simulink model "BLDC_FOC"  (R2020a)
settings: Solver=VariableStepAuto  StartTime=0.0  StopTime=2  RelTol=1e-3
InitFcn:
  | BLDC_FOC_Params
model workspace (MAT data in the model file):
  PhaseInductance = 0.001
  PhaseResistance = Simulink.Parameter
  PhaseResistance.Value = 0.03
  PhaseResistance.DataType = 'auto'
  PhaseResistance.Dimensions = [1 1]
values from neighbouring files (symbols this model uses):
  AlignmentDuration = 3 * TimeConstant_s    (= 0.2025)    [BLDC_FOC_Params.m]
  BatteryCapacityAh = 1.4    [BLDC_FOC_Params.m]
  BatteryCRating = 70    [BLDC_FOC_Params.m]
  BatteryVoltage = 1    [BLDC_FOC_Params.m]
  MaxCurrentDraw = (BatteryCapacityAh * BatteryCRating)/MotorCount    (= 98)    [BLDC_FOC_Params.m]
  MinimalOpenLoopSpeed_rpm = 100    [BLDC_FOC_Params.m]
  MotorCount = 1    [BLDC_FOC_Params.m]
  MotorKt = 0.00506    [BLDC_FOC_Params.m]
  MotorKv = 1890    [BLDC_FOC_Params.m]
  MotorPolePairs = 4    [BLDC_FOC_Params.m]
  MotorStatorTeeth = 0    [BLDC_FOC_Params.m]
  NominalTorque_Nm = 0.00183    [BLDC_FOC_Params.m]
  PhaseResistance_Ohm = DeltaToPhase(TerminalResistance_Ohm)    [BLDC_FOC_Params.m]
  PhaseSelfInductance_H = DeltaToPhase(TerminalInductance_H)    [BLDC_FOC_Params.m]
  RotorInertia_KgM2 = 0.00000011    (= 1.1e-07)    [BLDC_FOC_Params.m]
  Svpwm_freq_hz = 20000    [BLDC_FOC_Params.m]
undefined symbols (not defined in the file or in its folder): Down, Up
libraries: ee_lib x19, nesl_utility x14, fl_lib x12, eeTransforms x4, simulink x2, eePwmGenerator x1, powerlib_meascontrol x1
settings Model: Creator=enzoe  LastModifiedBy=enzoe

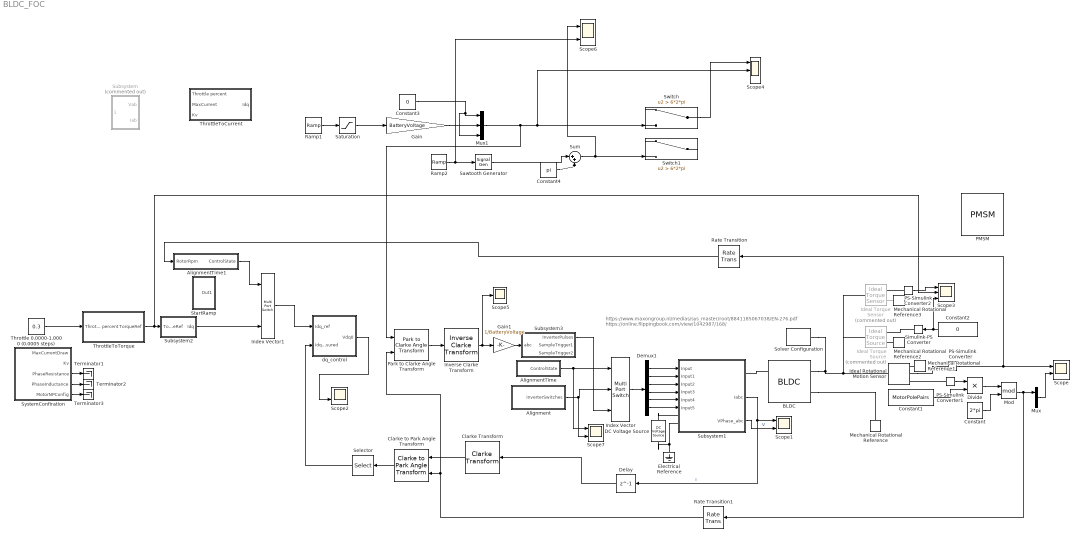
== system BLDC_FOC ==
  note: https://www.maxongroup.nl/medias/sys_master/root/8841185067038/EN-276.pdf
      | https://online.flippingbook.com/view/1042987/168/
  Alignment : Subsystem
  AlignmentTime : Subsystem
  AlignmentTime1 : Subsystem
  BLDC : ee_lib/Electromechanical/Permanent Magnet/BLDC  winding_type=ee.enum.statorconnection.wye  rotor_param=2  pm_flux_linkage=MaximumPermanentMagnetFluxLinkage Wb  theta_constant=pi / (MotorPolePairs*2) rad  emf_max=MaximumRotorInducedBackEmf_V V  DphiDtheta_tab=[0, -.1528, -.1528, .1528, .1528, 0] Wb/rad  back_emf_tab=[0, -9.6, -9.6, 9.6, 9.6, 0] V  rotor_angle_tab=[0, 7.5, 22.5, 37.5, 52.5, 60] deg  w_meas=RotorSpeedUsedForBackEmfMeasurement_RPM rpm  nPolePairs=MotorPolePairs  stator_param=ee.enum.statorparam.LsLmMs  machine_param=ee.enum.dqparameterization.constant  Ld=PhaseInductance H  Lq=PhaseInductance H  idVec=[-200, 0, 200] A  iqVec=[-200, 0, 200] A  LdMatrix=0.00022 * ones(3, 3) H  LqMatrix=0.00022 * ones(3, 3) H  L0=0.00016 H  Ls=PhaseSelfInductance_H H  Lm=StatorInductanceFluctuation_H H  Ms=StatorMutualInductance_H H  Rs=PhaseResistance_Ohm Ohm  zero_sequence=ee.enum.park.zerosequence.include  J=RotorInertia_KgM2 kg*m^2  lam=RotorDamping_NmRads N*m/(rad/s)  axes_param=2  i_d_specify=off  i_d_priority=None  i_d=0 A  i_d_nominal_specify=off  i_d_nominal_unit=A  i_d_nominal_value=1  i_q_specify=off  i_q_priority=None  i_q=0 A  i_q_nominal_specify=off  i_q_nominal_unit=A  i_q_nominal_value=1  torque_specify=off  torque_priority=None  torque=0 N*m  torque_nominal_specify=off  torque_nominal_unit=N*m  torque_nominal_value=1  angular_velocity_specify=off  angular_velocity_priority=High  angular_velocity=0 rpm  angular_velocity_nominal_specify=off  angular_velocity_nominal_unit=rpm  angular_velocity_nominal_value=1  angular_position_specify=off  angular_position_priority=High  angular_position=0 deg  angular_position_nominal_specify=off  angular_position_nominal_unit=deg  angular_position_nominal_value=1  loss_param=ee.enum.ironloss.none  losses_oc=[0, 0, 0] W  losses_sc=[0, 0, 0] W  f_losses=60 Hz  Isc_losses=95 A  Tmeas=298.15 K  alpha=3.93e-3 1/K  alpha_flux=-0.001 1/K  stator_thermal_mass=100 J/K  rotor_thermal_mass=200 J/K  Rm_percent_rotor=90  Rd_percent_rotor=30  temperatureA_specify=off  temperatureA_priority=High  temperatureA=25 degC  temperatureA_nominal_specify=off  temperatureA_nominal_unit=degC  temperatureA_nominal_value=1  temperatureB_specify=off  temperatureB_priority=High  temperatureB=25 degC  temperatureB_nominal_specify=off  temperatureB_nominal_unit=degC  temperatureB_nominal_value=1  temperatureC_specify=off  temperatureC_priority=High  temperatureC=25 degC  temperatureC_nominal_specify=off  temperatureC_nominal_unit=degC  temperatureC_nominal_value=1  temperatureR_specify=off  temperatureR_priority=High  temperatureR=25 degC  temperatureR_nominal_specify=off  temperatureR_nominal_unit=degC  temperatureR_nominal_value=1
      settings: SourceProductBaseCode=PS  InternalSimscapePortConfiguration="{\"Bottom\":[],\"Left\":[{\"id\":\"N\",\"label\":\"~\",\"type\":\"foundation.electrical.three_phase\"},{\"id\":\"n\",\"label\":\"n\",\"type\":\"foundation.electrical.electrical\"}],\"Right\":[{\"id\":\"R\",\"label\":\"R\",\"type\":\"foundation.mechanical.rotational.rotational\"},{\"id\":\"C\",\"label\":\"C\",\"type\":\"foundation.mechanical.rotational.rotational\"}],\"Top\":[]}"
  Clarke Transform : eeTransforms/Clarke Transform  PowerInvariant=off
      settings: SourceProductBaseCode=PS
  Clarke to Park Angle Transform : eeTransforms/Clarke to Park Angle Transform  AxisAlignment=D-axis
      settings: SourceProductBaseCode=PS
  Constant : Constant  Value=2*pi
  Constant1 : Constant  Value=MotorPolePairs
  Constant2 : Constant  Value=0
  Constant3 : Constant  Value=0
  Constant4 : Constant  Value=pi
  DC Voltage Source : ee_lib/Additional Components/SPICE Sources/DC Voltage Source  DC=BatteryVoltage V
  Delay : Delay  DelayLength=1
  Demux1 : Demux  Outputs=6
  Divide : Product  Inputs=**
  Electrical Reference : fl_lib/Electrical/Electrical Elements/Electrical Reference
  Gain : Gain  Gain=BatteryVoltage
  Gain1 : Gain  Gain=1/BatteryVoltage
  Ideal Rotational Motion Sensor : fl_lib/Mechanical/Mechanical Sensors/Ideal Rotational Motion Sensor  wrap_angle=simscape.enum.onoff.off  offset=0 rad
  Ideal Torque Sensor : fl_lib/Mechanical/Mechanical Sensors/Ideal Torque Sensor  Commented=on
  Ideal Torque Source : fl_lib/Mechanical/Mechanical Sources/Ideal Torque Source  Commented=on
  Index Vector : MultiPortSwitch  DataPortOrder=Zero-based contiguous  Inputs=2  zeroidx=on
  Index Vector1 : MultiPortSwitch  DataPortOrder=Zero-based contiguous  Inputs=2  zeroidx=on
  Inverse Clarke Transform : eeTransforms/Inverse Clarke Transform  PowerInvariant=off
      settings: SourceProductBaseCode=PS
  Mechanical Rotational Reference{,1..3} (4 alike) : fl_lib/Mechanical/Rotational Elements/Mechanical Rotational Reference
  Mod : Math  Operator=mod  SaturateOnIntegerOverflow=on
  Mux : Mux  Inputs=2
  Mux1 : Mux  Inputs=3
  PMSM : ee_lib/Electromechanical/Permanent Magnet/PMSM  winding_type=ee.enum.statorconnection.wye  machine_param=ee.enum.pmsm.parameterization.constant  nPolePairs=MotorPolePairs  pmflux_param=ee.enum.pmflux.backemfconstant  pm_flux_linkage=0.03 Wb  torque_constant=0.18 N*m/A  back_emf_constant=BackEmfConstant_VRpm V/rpm  stator_param=ee.enum.statorparam.LsLmMs  Ld=0.00019 H  Lq=0.00025 H  idVec=[-200, 0, 200] A  iqVec=[-200, 0, 200] A  LdMatrix=0.0002 * ones(3, 3) H  LqMatrix=0.0002 * ones(3, 3) H  PmMatrix=0.1 * ones(3, 3) Wb  ktMatrix=0.18 * ones(3, 3) N*m/A  keMatrix=0.18 * ones(3, 3) V/(rad/s)  L0=0.00016 H  Ls=PhaseSelfInductance_H H  Lm=StatorInductanceFluctuation_H H  Ms=StatorMutualInductance_H H  Rs=PhaseResistance_Ohm Ohm  zero_sequence=ee.enum.park.zerosequence.include  J=RotorInertia_KgM2 kg*m^2  lam=RotorDamping_NmRads N*m/(rad/s)  axes_param=ee.enum.rotorangle.daxis  i_d_specify=off  i_d_priority=None  i_d=0 A  i_d_nominal_specify=off  i_d_nominal_unit=A  i_d_nominal_value=1  i_q_specify=off  i_q_priority=None  i_q=0 A  i_q_nominal_specify=off  i_q_nominal_unit=A  i_q_nominal_value=1  torque_specify=off  torque_priority=None  torque=0 N*m  torque_nominal_specify=off  torque_nominal_unit=N*m  torque_nominal_value=1  angular_velocity_specify=off  angular_velocity_priority=High  angular_velocity=0 rpm  angular_velocity_nominal_specify=off  angular_velocity_nominal_unit=rpm  angular_velocity_nominal_value=1  angular_position_specify=off  angular_position_priority=High  angular_position=0 deg  angular_position_nominal_specify=off  angular_position_nominal_unit=deg  angular_position_nominal_value=1  loss_param=ee.enum.ironloss.none  losses_oc=[0, 0, 0] W  losses_sc=[0, 0, 0] W  f_losses=60 Hz  Isc_losses=95 A  Tmeas=298.15 K  alpha=3.93e-3 1/K  alpha_flux=-0.001 1/K  stator_thermal_mass=100 J/K  rotor_thermal_mass=200 J/K  Rm_percent_rotor=90  Rd_percent_rotor=30  temperatureA_specify=off  temperatureA_priority=High  temperatureA=25 degC  temperatureA_nominal_specify=off  temperatureA_nominal_unit=degC  temperatureA_nominal_value=1  temperatureB_specify=off  temperatureB_priority=High  temperatureB=25 degC  temperatureB_nominal_specify=off  temperatureB_nominal_unit=degC  temperatureB_nominal_value=1  temperatureC_specify=off  temperatureC_priority=High  temperatureC=25 degC  temperatureC_nominal_specify=off  temperatureC_nominal_unit=degC  temperatureC_nominal_value=1  temperatureR_specify=off  temperatureR_priority=High  temperatureR=25 degC  temperatureR_nominal_specify=off  temperatureR_nominal_unit=degC  temperatureR_nominal_value=1
      settings: InternalSimscapePortConfiguration="{\"Bottom\":[],\"Left\":[{\"id\":\"N\",\"label\":\"~\",\"type\":\"foundation.electrical.three_phase\"},{\"id\":\"n\",\"label\":\"n\",\"type\":\"foundation.electrical.electrical\"}],\"Right\":[{\"id\":\"R\",\"label\":\"R\",\"type\":\"foundation.mechanical.rotational.rotational\"},{\"id\":\"C\",\"label\":\"C\",\"type\":\"foundation.mechanical.rotational.rotational\"}],\"Top\":[]}"
  PS-Simulink Converter : nesl_utility/PS-Simulink Converter  PhysicalDomain=network_engine_domain  SubClassName=ps_output  LeftPortType=input  RightPortType=output  PseudoPeriodic=off  Frequencies=[]  Unit=inherit  AffineConversion=off
  PS-Simulink Converter1 : nesl_utility/PS-Simulink Converter  PhysicalDomain=network_engine_domain  SubClassName=ps_output  LeftPortType=input  RightPortType=output  PseudoPeriodic=off  Frequencies=[]  Unit=inherit  AffineConversion=off
  PS-Simulink Converter2 : nesl_utility/PS-Simulink Converter  PhysicalDomain=network_engine_domain  SubClassName=ps_output  LeftPortType=input  RightPortType=output  PseudoPeriodic=off  Frequencies=[]  Unit=inherit  AffineConversion=off
  Park to Clarke Angle Transform : eeTransforms/Park to Clarke Angle Transform  AxisAlignment=D-axis
      settings: SourceProductBaseCode=PS
  Ramp1 : simulink/Sources/Ramp  slope=2  start=0  InitialOutput=0
  Ramp2 : simulink/Sources/Ramp  slope=-2  start=0  InitialOutput=2
  Rate Transition : RateTransition
  Rate Transition1 : RateTransition
  Saturation : Saturate  UpperLimit=1  LowerLimit=0
  Sawtooth Generator : SignalGenerator  WaveForm=sawtooth  TimeSource=Use external signal  Amplitude=pi  Frequency=20*pi  Units=rad/sec
  Scope{,1..2,6..7} (5 alike) : Scope  NumInputPorts=2
  Scope3 : Scope  NumInputPorts=3
  Scope4 : Scope  NumInputPorts=3
  Scope5 : Scope
  Selector : Selector  InputPortWidth=3  IndexOptions=Index vector (dialog)  Indices=[1 2]  OutputSizes=1
  Simulink-PS Converter : nesl_utility/Simulink-PS Converter  PhysicalDomain=network_engine_domain  SubClassName=ps_input  LeftPortType=input  RightPortType=output  PseudoPeriodic=off  Frequencies=[]  NoiseDistribution=none  NoiseParameters=[]  Unit=1  AffineConversion=off  FilteringAndDerivatives=provide  SimscapeFilterOrder=1  InputFilterTimeConstant=0.001  UdotUserProvided=0
  Solver Configuration : nesl_utility/Solver Configuration  PhysicalDomain=network_engine_domain  SubClassName=solver  LeftPortType=input  RightPortType=generic  Tones=[]  Harmonics=[]  SimulateNoise=off  Profile=off  UseLocalSampling=off  EnableSwitchedLinearOptims=on  FrequencyDomain=off  UseCCode=off  RelTol=0.001  AbsTol=1e-06  MinStep=1e-09  ToWorkspace=off  RevertToSquareIcSolve=off  NumHomotopyIterations=100  PhasorMode=off  PhasorModeNumHarmonics=1  DoDC=off  ResidualTolerance=1e-09  UseLocalSolver=on  LocalSolverChoice=NE_BACKWARD_EULER_ADVANCER  LocalSolverSampleTime=1e-4  DoFixedCost=on  MaxNonlinIter=3  MaxModeIter=2  LinearAlgebra=auto  EquationFormulation=NE_TIME_EF  DelaysMemoryBudget=1024  AutomaticFiltering=on  FilteringTimeConstant=0.001  PartitionStorageMethod=AS_NEEDED  PartitionMemoryBudget=1024  PartitionMethod=ROBUST
  StartRamp : Subsystem
  Subsystem : Subsystem  Commented=on
  Subsystem1 : Subsystem
      settings: PortSchema="{\"entries\":[{\"content\":{\"sides\":[{\"content\":{\"connectorIds\":[\"In1\",\"In2\",\"In3\",\"In4\",\"In5\",\"In6\",\"LConn1\",\"LConn2\"]},\"type\":\"ConnectorPlacement.EquallySpacedRectSide\",\"uuid\":\"4a91dc72-3770-4abf-bed3-c4a9f6b4b65e\"},{\"content\":{\"connectorIds\":[\"RConn1\",\"Out1\",\"Out2\"],\"side\":\"RIGHT\"},\"type\":\"ConnectorPlacement.EquallySpacedRectSide\",\"uuid\":\"c06ed33e-65a1-40a2-85db-2ae3e949e0d2\"},{\"content\":{\"connectorIds\":[],\"side\":\"TOP\"},\"type\":\"ConnectorPlacement.EquallySpacedRectSide\",\"uuid\":\"0b7af1c1-9cb6-4ccc-8dcc-bc330691322d\"}]},\"type\":\"ConnectorPlacement.EquallySpacedConnector\",\"uuid\":\"fc3d9dc5-347b-4e6e-ad3c-0830f77ecff8\"}],\"packageUris\":[\"http://schema.mathworks.com/mf0/Connector/19700101\"],\"version\":\"1.0\"}"
  Subsystem2 : Subsystem
  Subsystem3 : Subsystem
  Sum : Sum  Inputs=|++
  Switch : Switch  Criteria=u2 > Threshold  Threshold=6*2*pi
  Switch1 : Switch  Criteria=u2 > Threshold  Threshold=6*2*pi
  SystemConfiration : Subsystem
  Terminator1 : Terminator
  Terminator2 : Terminator
  Terminator3 : Terminator
  Throttle 0.0000-1.0000 (0.0005 steps) : Constant  Value=0.3
  ThrottleToCurrent : Subsystem
  ThrottleToTorque : Subsystem
  dq_control : Subsystem
  wires:
  Clarke to Park Angle Transform/1 -> Selector/1
  Selector/1 -> dq_control/2(Idq_measured)
  Clarke Transform/1 -> Clarke to Park Angle Transform/1
  Demux1/1 -> Subsystem1/1(Input)
  Demux1/2 -> Subsystem1/2(Input1)
  Demux1/3 -> Subsystem1/3(Input2)
  Demux1/4 -> Subsystem1/4(Input3)
  Demux1/6 -> Subsystem1/6(Input5)
  PS-Simulink Converter/1 -> Rate Transition/1, Scope/1
  Delay/1 -> Clarke Transform/1
  SystemConfiration/3(PhaseResistance) -> Terminator1/1
  SystemConfiration/4(PhaseInductance) -> Terminator2/1
  SystemConfiration/5(MotorNPConfig) -> Terminator3/1
  Constant/1 -> Mod/2
  Subsystem1/1(Iabc) -> Delay/1, Scope1/1  "I"
  Demux1/5 -> Subsystem1/5(Input4)
  Mod/1 -> Rate Transition1/1, Mux/1
  PS-Simulink Converter1/1 -> Divide/1
  Constant1/1 -> Divide/2
  Divide/1 -> Mod/1
  Park to Clarke Angle Transform/1 -> Inverse Clarke Transform/1
  Gain1/1 -> Subsystem3/1(abc)
  Mux/1 -> Scope/2
  Subsystem1/2(VPhase_abc) -> Scope1/2  "V"
  Constant2/1 -> Scope3/3, Simulink-PS Converter/1
  PS-Simulink Converter2/1 -> Scope3/1
  ThrottleToTorque/1(TorqueRef) -> Scope3/2, Subsystem2/1(TorqueRef)
  Switch/1 -> Scope4/1
  Constant3/1 -> Mux1/3, Mux1/1
  Mux1/1 -> Park to Clarke Angle Transform/1, Switch/3, Scope4/2
  Gain/1 -> Mux1/2
  dq_control/1(Vdq0) -> Scope2/2
  Inverse Clarke Transform/1 -> Gain1/1, Scope5/1
  Ramp1/1 -> Saturation/1
  Saturation/1 -> Gain/1
  Sawtooth Generator/1 -> Sum/1
  Constant4/1 -> Sum/2
  Sum/1 -> Scope6/1, Switch1/3
  Throttle 0.0000-1.0000 (0.0005 steps)/1 -> ThrottleToTorque/1(Throttle percent)
  Ramp2/1 -> Sawtooth Generator/1, Scope6/2
  Alignment/1(InverterSwitches) -> Scope7/2, Index Vector/2
  Index Vector/1 -> Demux1/1
  Subsystem3/1(InverterPulses) -> Index Vector/3
  AlignmentTime/1(ControlState) -> Scope7/1, Index Vector/1
  Rate Transition1/1 -> Clarke to Park Angle Transform/2, Park to Clarke Angle Transform/2
  AlignmentTime1/1(ControlState) -> Index Vector1/1
  Subsystem2/1(Idq) -> Index Vector1/3
  Index Vector1/1 -> dq_control/1(Idq_ref)
  Rate Transition/1 -> AlignmentTime1/1(RotorRpm)
  connections:
  DC Voltage Source/LConn1 -- Subsystem1/LConn1
  DC Voltage Source/RConn1 -- Electrical Reference/LConn1 -- Subsystem1/LConn2
  BLDC/RConn2 -- Mechanical Rotational Reference/LConn1
  Solver Configuration/RConn1 -- BLDC/RConn1 -- Ideal Torque Source/LConn1 -- Ideal Torque Sensor/LConn1 -- Ideal Rotational Motion Sensor/LConn1
  Ideal Rotational Motion Sensor/RConn2 -- PS-Simulink Converter/LConn1
  PS-Simulink Converter1/LConn1 -- Ideal Rotational Motion Sensor/RConn3
  Ideal Rotational Motion Sensor/RConn1 -- Mechanical Rotational Reference1/LConn1
  BLDC/LConn1 -- Subsystem1/RConn1
  Mechanical Rotational Reference2/LConn1 -- Ideal Torque Source/RConn2
  Simulink-PS Converter/RConn1 -- Ideal Torque Source/RConn1
  PS-Simulink Converter2/LConn1 -- Ideal Torque Sensor/RConn2
  Ideal Torque Sensor/RConn1 -- Mechanical Rotational Reference3/LConn1

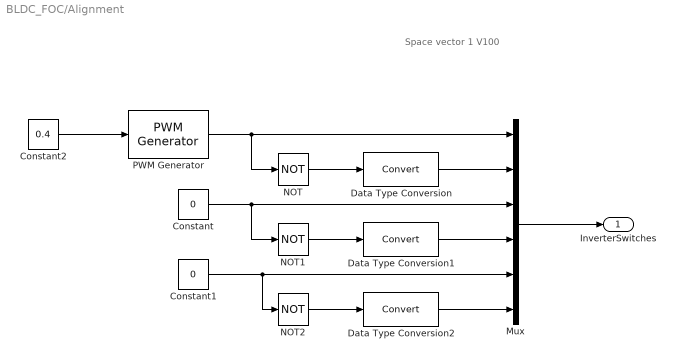
== system BLDC_FOC/Alignment ==
  note: Space vector 1
      | V100
  Constant : Constant  Value=0
  Constant1 : Constant  Value=0
  Constant2 : Constant  Value=0.4
  Data Type Conversion : DataTypeConversion
  Data Type Conversion1 : DataTypeConversion
  Data Type Conversion2 : DataTypeConversion
  Mux : Mux  Inputs=6
  NOT : Logic  Operator=NOT  IconShape=distinctive  AllPortsSameDT=off  OutDataTypeStr=boolean
  NOT1 : Logic  Operator=NOT  IconShape=distinctive  AllPortsSameDT=off  OutDataTypeStr=boolean
  NOT2 : Logic  Operator=NOT  IconShape=distinctive  AllPortsSameDT=off  OutDataTypeStr=boolean
  PWM Generator : eePwmGenerator/PWM Generator  CarrCount=Up-Down  Tper=1/Svpwm_freq_hz  Ts=0
  InverterSwitches : Outport
  wires:
  Mux/1 -> InverterSwitches/1
  Constant/1 -> Mux/3, NOT1/1
  NOT/1 -> Data Type Conversion/1
  NOT1/1 -> Data Type Conversion1/1
  Constant1/1 -> NOT2/1, Mux/5
  Constant2/1 -> PWM Generator/1
  Data Type Conversion/1 -> Mux/2
  Data Type Conversion1/1 -> Mux/4
  NOT2/1 -> Data Type Conversion2/1
  Data Type Conversion2/1 -> Mux/6
  PWM Generator/1 -> NOT/1, Mux/1

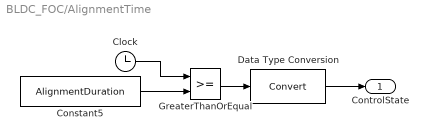
== system BLDC_FOC/AlignmentTime ==
  Clock : Clock
      settings: Decimation=100
  Constant5 : Constant  Value=AlignmentDuration
  Data Type Conversion : DataTypeConversion
  GreaterThanOrEqual : RelationalOperator  OutDataTypeStr=boolean  RndMeth=Simplest
  ControlState : Outport
  wires:
  GreaterThanOrEqual/1 -> Data Type Conversion/1
  Clock/1 -> GreaterThanOrEqual/1
  Constant5/1 -> GreaterThanOrEqual/2
  Data Type Conversion/1 -> ControlState/1

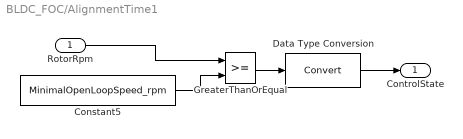
== system BLDC_FOC/AlignmentTime1 ==
  RotorRpm : Inport
  Constant5 : Constant  Value=MinimalOpenLoopSpeed_rpm
  Data Type Conversion : DataTypeConversion
  GreaterThanOrEqual : RelationalOperator  OutDataTypeStr=boolean  RndMeth=Simplest
  ControlState : Outport
  wires:
  Data Type Conversion/1 -> ControlState/1
  Constant5/1 -> GreaterThanOrEqual/2
  RotorRpm/1 -> GreaterThanOrEqual/1
  GreaterThanOrEqual/1 -> Data Type Conversion/1

== system BLDC_FOC/StartRamp ==
  Out1 : Outport

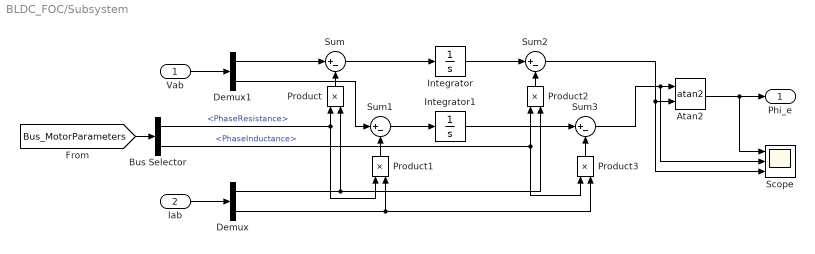
== system BLDC_FOC/Subsystem ==
  Vab : Inport
  Iab : Inport  Port=2
  Atan2 : Trigonometry  Operator=atan2
  Bus Selector : BusSelector  OutputSignals=PhaseResistance,PhaseInductance
  Demux : Demux  Outputs=2
  Demux1 : Demux  Outputs=2
  Integrator : Integrator
  Integrator1 : Integrator
  Product{,1..3} (4 alike) : Product
  Scope : Scope  NumInputPorts=3
  Sum{,1..3} (4 alike) : Sum  Inputs=|+-
  Phi_e : Outport
  wires:
  Iab/1 -> Demux/1
  Vab/1 -> Demux1/1
  Demux1/1 -> Sum/1
  Demux/1 -> Product/2, Product2/2
  [Bus_MotorParameters] -> Bus Selector/1
  Bus Selector/1 -> Product1/1, Product/1  "<PhaseResistance>"
  Product/1 -> Sum/2
  Product1/1 -> Sum1/2
  Demux1/2 -> Sum1/1
  Demux/2 -> Product3/2, Product1/2
  Sum/1 -> Integrator/1
  Sum1/1 -> Integrator1/1
  Integrator/1 -> Sum2/1
  Integrator1/1 -> Sum3/1
  Sum2/1 -> Scope/3, Atan2/2
  Sum3/1 -> Scope/2, Atan2/1
  Product2/1 -> Sum2/2
  Product3/1 -> Sum3/2
  Bus Selector/2 -> Product3/1, Product2/1  "<PhaseInductance>"
  Atan2/1 -> Scope/1, Phi_e/1

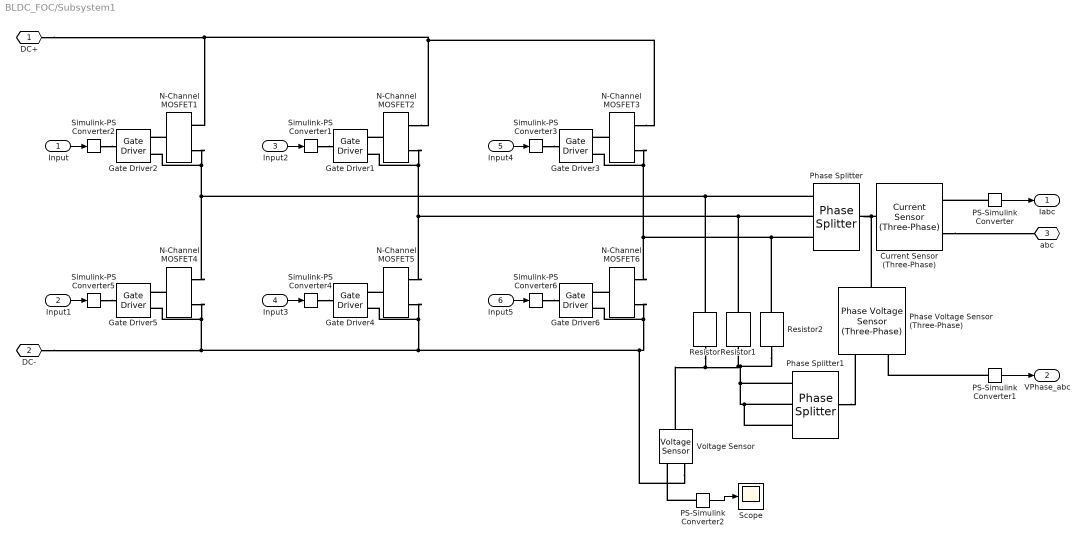
== system BLDC_FOC/Subsystem1 ==
  Input : Inport
  Input1 : Inport  Port=2
  Input2 : Inport  Port=3
  Input3 : Inport  Port=4
  Input4 : Inport  Port=5
  Input5 : Inport  Port=6
  Current Sensor (Three-Phase) : ee_lib/Sensors & Transducers/Current Sensor (Three-Phase)
  Gate Driver{1..6} (6 alike) : ee_lib/Semiconductors & Converters/Gate Driver  vHigh=15 V  vLow=0 V  parameterization=1  rHigh=2 Ohm  rLow=2 Ohm  tRise=20 ns  tFall=20 ns  cLoad=10 nF  enable_faults=0  t_fault=1 s  fault_type=1  uHighValue=0.7  uLowValue=0.3  tHigh=50 ns  tLow=50 ns  ZonTime_specify=off  ZonTime_priority=None  ZonTime=0 s  ZoffTime_specify=off  ZoffTime_priority=None  ZoffTime=0 s  uHigh=2.0 V  uLow=0.8 V
      settings: SourceProductBaseCode=PS  InternalSimscapePortConfiguration="{\"Bottom\":[],\"Left\":[{\"id\":\"u\",\"label\":\"u\",\"type\":\"input\"}],\"Right\":[{\"id\":\"G\",\"label\":\"G\",\"type\":\"foundation.electrical.electrical\"},{\"id\":\"S\",\"label\":\"S\",\"type\":\"foundation.electrical.electrical\"}],\"Top\":[]}"
  N-Channel MOSFET{1..6} (6 alike) : ee_lib/Semiconductors & Converters/N-Channel MOSFET  paramTerminal=ee.enum.mosfet.numberOfTerminals.three  parameterization=ee.enum.parameterization.datasheet  prmDatasheet=ee.enum.temperatureParameterization.none  prmEquCoeff=ee.enum.temperatureParameterization.none  Beta=5.0 A/V^2  Rds=0.025 Ohm  Id=6.0 A  Vgs=10 V  Vth=1.7 V  Vth0=1.7 V  lam=0 1/V  gamma_vth=0.5 V^0.50000  phib=0.5 V  Vth1=1.9071 V  Vbs1=-1 V  Vth2=2.066 V  Vbs2=-2 V  Tmeas=25 degC  RS=0.0001 Ohm  RD=0.01 Ohm  RB=0.001 Ohm  C_param=ee.enum.mosfet.capacitanceParam.fixedciss  C_GS=270 pF  C_GD=80 pF  C_DS=0 pF  C_iss=350 pF  C_rss=80 pF  C_oss=0 pF  charge_linearity_param=ee.enum.mosfet.cgdLinearity.constant  C_OX=200 pF  V_C_OX=-0.5 V  C_iss_vec=[720, 700, 590, 470, 390, 310] pF  C_rss_vec=[450, 400, 300, 190, 95, 55] pF  C_oss_vec=[900, 810, 690, 420, 270, 170] pF  C_GS_vec=[270, 300, 290, 280, 295, 255] pF  C_GD_vec=[450, 400, 300, 190, 95, 55] pF  C_DS_vec=[450, 410, 390, 230, 175, 115] pF  C_Vds_vec=[.1, .3, 1, 3, 10, 30] V  V_GS_for_cap_data=0 V  charge_linearity_param_vgb=ee.enum.mosfet.cgbLinearity.instantly  IsDiode=0 A  Vbi=0.6 V  n=1  Cj0Diode=0 pF  TT=50e-9 s  dVth_dT=-6 mV/K  dVth0_dT=-6 mV/K  Rds_T2=0.037 Ohm  Tmeas2=125 degC  BEXDatasheet=-1.5  BEXEquCoeff=-1.5  etaisDatasheet=3  etaisEquCoeff=3  TdeviceDatasheet=25 degC  TdeviceEquCoeff=25 degC  thermal_network_parameterization=ee.enum.thermalNetworkTopology.cauer  Rth=[0, 10] K/W  Rth_Foster=[4, 6] K/W  thermal_mass_parameterization=ee.enum.thermalNetwork.timeconstant  thermal_mass=[0, 1] J/K  thermal_mass_Foster=[1.5, 3] J/K  thermal_time_constant=[0, 10] s  thermal_time_constant_Foster=[6, 18] s  thermal_mass_initial_temperatures=[25, 25] degC  betaref=18 A/V^2  Vfbref=-1.1 V  gamma=3.5 V^0.50000  phib2ref=1 V  thesatref=0.4 1/V  alpha=0  Vp=5e-2 V  thesrref=0 1/V  m=8  Tref=25 degC  Cox=1500 pF  Cgso=100 pF  Cgdo=14 pF  Rsref=2e-3 Ohm  Rdref=0.17 Ohm  Rgref=8.4 Ohm  Rbref=2e-3 Ohm  Isref=5.2e-13 A  Cj0=480 pF  Tprm=1  etabet=1.3  Stvfb=5e-4 V/K  Stphib=-8.5e-4 V/K  etasat=1.04  etasr=0.65  etar=0.95  etais=3  Tsim=25 degC  T0=[25, 25] degC
  PS-Simulink Converter : nesl_utility/PS-Simulink Converter  PhysicalDomain=network_engine_domain  SubClassName=ps_output  LeftPortType=input  RightPortType=output  PseudoPeriodic=off  Frequencies=[]  Unit=inherit  AffineConversion=off
  PS-Simulink Converter1 : nesl_utility/PS-Simulink Converter  PhysicalDomain=network_engine_domain  SubClassName=ps_output  LeftPortType=input  RightPortType=output  PseudoPeriodic=off  Frequencies=[]  Unit=inherit  AffineConversion=off
  PS-Simulink Converter2 : nesl_utility/PS-Simulink Converter  PhysicalDomain=network_engine_domain  SubClassName=ps_output  LeftPortType=input  RightPortType=output  PseudoPeriodic=off  Frequencies=[]  Unit=inherit  AffineConversion=off
  Phase Splitter : ee_lib/Connectors & References/Phase Splitter
      settings: SourceProductBaseCode=PS
  Phase Splitter1 : ee_lib/Connectors & References/Phase Splitter
      settings: SourceProductBaseCode=PS
  Phase Voltage Sensor (Three-Phase) : ee_lib/Sensors & Transducers/Phase Voltage Sensor (Three-Phase)
      settings: SourceProductBaseCode=PS
  Resistor : fl_lib/Electrical/Electrical Elements/Resistor  R=1000 Ohm  i_specify=off  i_priority=None  i=0 A  i_nominal_specify=off  i_nominal_unit=A  i_nominal_value=1  v_specify=off  v_priority=None  v=0 V  v_nominal_specify=off  v_nominal_unit=V  v_nominal_value=1
  Resistor1 : fl_lib/Electrical/Electrical Elements/Resistor  R=1000 Ohm  i_specify=off  i_priority=None  i=0 A  i_nominal_specify=off  i_nominal_unit=A  i_nominal_value=1  v_specify=off  v_priority=None  v=0 V  v_nominal_specify=off  v_nominal_unit=V  v_nominal_value=1
  Resistor2 : fl_lib/Electrical/Electrical Elements/Resistor  R=1000 Ohm  i_specify=off  i_priority=None  i=0 A  i_nominal_specify=off  i_nominal_unit=A  i_nominal_value=1  v_specify=off  v_priority=None  v=0 V  v_nominal_specify=off  v_nominal_unit=V  v_nominal_value=1
  Scope : Scope
  Simulink-PS Converter{1..6} (6 alike) : nesl_utility/Simulink-PS Converter  PhysicalDomain=network_engine_domain  SubClassName=ps_input  LeftPortType=input  RightPortType=output  PseudoPeriodic=off  Frequencies=[]  NoiseDistribution=none  NoiseParameters=[]  Unit=1  AffineConversion=off  FilteringAndDerivatives=provide  SimscapeFilterOrder=1  InputFilterTimeConstant=0.001  UdotUserProvided=0
  Voltage Sensor : fl_lib/Electrical/Electrical Sensors/Voltage Sensor
  DC+ : PMIOPort  Side=Left
  DC- : PMIOPort  Port=2  Side=Left
  abc : PMIOPort  Port=3  Side=Right
  Iabc : Outport
  VPhase_abc : Outport  Port=2
  wires:
  Input/1 -> Simulink-PS Converter2/1
  Input1/1 -> Simulink-PS Converter5/1
  Input2/1 -> Simulink-PS Converter1/1
  Input3/1 -> Simulink-PS Converter4/1
  Input4/1 -> Simulink-PS Converter3/1
  Input5/1 -> Simulink-PS Converter6/1
  PS-Simulink Converter/1 -> Iabc/1
  PS-Simulink Converter1/1 -> VPhase_abc/1
  PS-Simulink Converter2/1 -> Scope/1
  connections:
  N-Channel MOSFET1/LConn1 -- Gate Driver2/RConn1
  N-Channel MOSFET1/RConn2 -- Resistor/LConn1 -- Phase Splitter/RConn1 -- N-Channel MOSFET4/RConn1 -- Gate Driver2/RConn2
  Simulink-PS Converter2/RConn1 -- Gate Driver2/LConn1
  Simulink-PS Converter1/RConn1 -- Gate Driver1/LConn1
  N-Channel MOSFET2/RConn2 -- Resistor1/LConn1 -- Phase Splitter/RConn2 -- N-Channel MOSFET5/RConn1 -- Gate Driver1/RConn2
  N-Channel MOSFET2/LConn1 -- Gate Driver1/RConn1
  N-Channel MOSFET3/LConn1 -- Gate Driver3/RConn1
  N-Channel MOSFET3/RConn2 -- Resistor2/LConn1 -- Phase Splitter/RConn3 -- N-Channel MOSFET6/RConn1 -- Gate Driver3/RConn2
  Simulink-PS Converter3/RConn1 -- Gate Driver3/LConn1
  Simulink-PS Converter6/RConn1 -- Gate Driver6/LConn1
  Simulink-PS Converter4/RConn1 -- Gate Driver4/LConn1
  Simulink-PS Converter5/RConn1 -- Gate Driver5/LConn1
  N-Channel MOSFET6/LConn1 -- Gate Driver6/RConn1
  N-Channel MOSFET6/RConn2 -- DC-/RConn1 -- N-Channel MOSFET4/RConn2 -- Gate Driver5/RConn2 -- N-Channel MOSFET5/RConn2 -- Gate Driver4/RConn2 -- Voltage Sensor/RConn2 -- Gate Driver6/RConn2
  N-Channel MOSFET5/LConn1 -- Gate Driver4/RConn1
  N-Channel MOSFET4/LConn1 -- Gate Driver5/RConn1
  DC+/RConn1 -- N-Channel MOSFET3/RConn1 -- N-Channel MOSFET2/RConn1 -- N-Channel MOSFET1/RConn1
  Current Sensor (Three-Phase)/RConn2 -- abc/RConn1
  Current Sensor (Three-Phase)/LConn1 -- Phase Voltage Sensor (Three-Phase)/LConn1 -- Phase Splitter/LConn1
  PS-Simulink Converter/LConn1 -- Current Sensor (Three-Phase)/RConn1
  Resistor/RConn1 -- Phase Splitter1/RConn3 -- Phase Splitter1/RConn2 -- Phase Splitter1/RConn1 -- Resistor2/RConn1 -- Resistor1/RConn1 -- Voltage Sensor/LConn1
  PS-Simulink Converter1/LConn1 -- Phase Voltage Sensor (Three-Phase)/RConn1
  Phase Splitter1/LConn1 -- Phase Voltage Sensor (Three-Phase)/RConn2
  PS-Simulink Converter2/LConn1 -- Voltage Sensor/RConn1

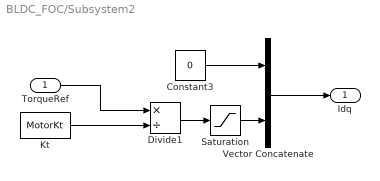
== system BLDC_FOC/Subsystem2 ==
  TorqueRef : Inport
  Constant3 : Constant  Value=0
  Divide1 : Product  Inputs=*/
  Kt : Constant  Value=MotorKt
  Saturation : Saturate  UpperLimit=2  LowerLimit=0
  Vector Concatenate : Concatenate
  Idq : Outport
  wires:
  Constant3/1 -> Vector Concatenate/1
  TorqueRef/1 -> Divide1/1
  Vector Concatenate/1 -> Idq/1
  Saturation/1 -> Vector Concatenate/2
  Divide1/1 -> Saturation/1
  Kt/1 -> Divide1/2

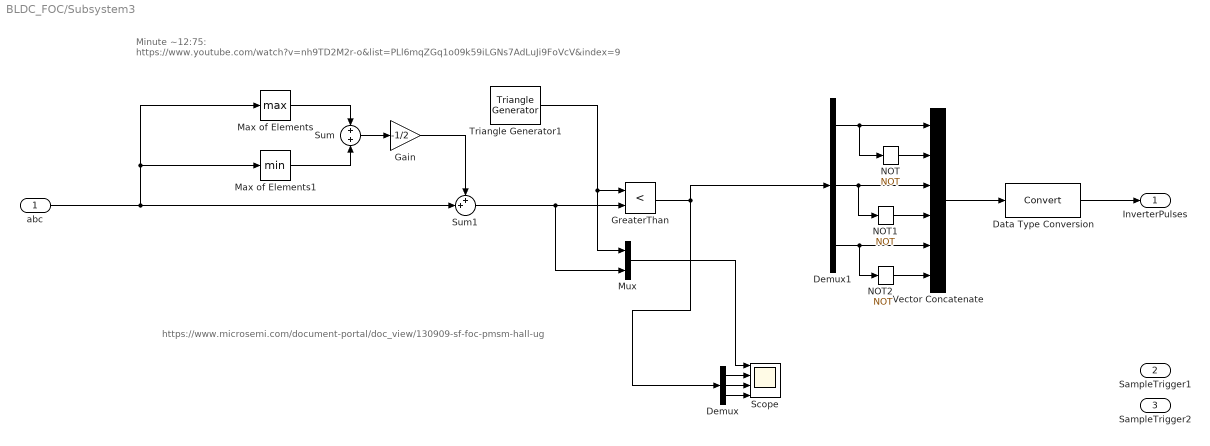
== system BLDC_FOC/Subsystem3 ==
  note: https://www.microsemi.com/document-portal/doc_view/130909-sf-foc-pmsm-hall-ug
  note: Minute ~12:75:
      | https://www.youtube.com/watch?v=nh9TD2M2r-o&list=PLl6mqZGq1o09k59iLGNs7AdLuJi9FoVcV&index=9
  abc : Inport
  Data Type Conversion : DataTypeConversion
  Demux : Demux  Outputs=3
  Demux1 : Demux  Outputs=3
  Gain : Gain  Gain=-1/2
  GreaterThan : RelationalOperator  Operator=<  OutDataTypeStr=boolean  RndMeth=Simplest
  Max of Elements : MinMax  Function=max
  Max of Elements1 : MinMax
  Mux : Mux  Inputs=2
  NOT : Logic  Operator=NOT  IconShape=distinctive  AllPortsSameDT=off  OutDataTypeStr=boolean
  NOT1 : Logic  Operator=NOT  IconShape=distinctive  AllPortsSameDT=off  OutDataTypeStr=boolean
  NOT2 : Logic  Operator=NOT  IconShape=distinctive  AllPortsSameDT=off  OutDataTypeStr=boolean
  Scope : Scope  NumInputPorts=4
  Sum : Sum  Inputs=+|+
  Sum1 : Sum  Inputs=++|
  Triangle Generator1 : powerlib_meascontrol/Pulse & Signal Generators/Triangle Generator  Freq=Svpwm_freq_hz  Phase=180  Ts=0
  Vector Concatenate : Concatenate  NumInputs=6
  InverterPulses : Outport
  SampleTrigger1 : Outport  Port=2
  SampleTrigger2 : Outport  Port=3
  wires:
  abc/1 -> Sum1/2, Max of Elements1/1, Max of Elements/1
  Sum1/1 -> Mux/2, GreaterThan/2
  Max of Elements1/1 -> Sum/2
  Sum/1 -> Gain/1
  Max of Elements/1 -> Sum/1
  Triangle Generator1/1 -> Mux/1, GreaterThan/1
  Mux/1 -> Scope/1
  GreaterThan/1 -> Demux/1, Demux1/1
  Demux/1 -> Scope/2
  Demux/2 -> Scope/3
  Demux/3 -> Scope/4
  NOT/1 -> Vector Concatenate/2
  NOT1/1 -> Vector Concatenate/4
  NOT2/1 -> Vector Concatenate/6
  Demux1/1 -> Vector Concatenate/1, NOT/1
  Demux1/3 -> Vector Concatenate/5, NOT2/1
  Demux1/2 -> Vector Concatenate/3, NOT1/1
  Vector Concatenate/1 -> Data Type Conversion/1
  Data Type Conversion/1 -> InverterPulses/1
  Gain/1 -> Sum1/1

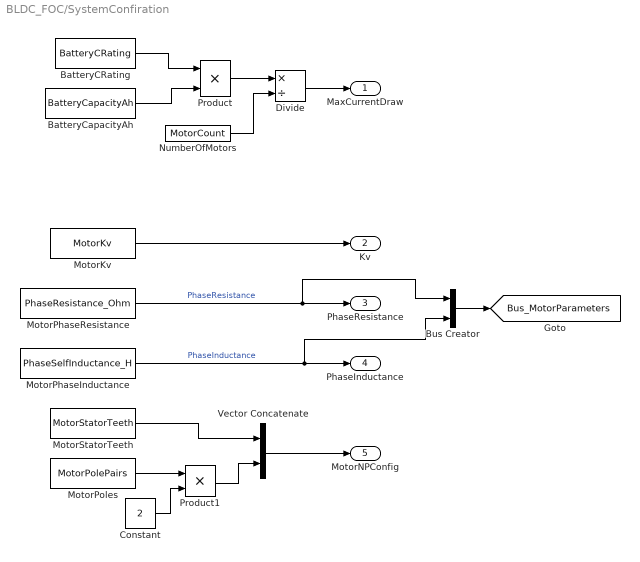
== system BLDC_FOC/SystemConfiration ==
  BatteryCRating : Constant  Value=BatteryCRating
  BatteryCapacityAh : Constant  Value=BatteryCapacityAh
  Bus Creator : BusCreator  Inputs=2
  Constant : Constant  Value=2
  Divide : Product  Inputs=*/
  MotorKv : Constant  Value=MotorKv
  MotorPhaseInductance : Constant  Value=PhaseSelfInductance_H
  MotorPhaseResistance : Constant  Value=PhaseResistance_Ohm
  MotorPoles : Constant  Value=MotorPolePairs
  MotorStatorTeeth : Constant  Value=MotorStatorTeeth
  NumberOfMotors : Constant  Value=MotorCount
  Product : Product
  Product1 : Product
  Vector Concatenate : Concatenate
  MaxCurrentDraw : Outport
  Kv : Outport  Port=2
  PhaseResistance : Outport  Port=3
  PhaseInductance : Outport  Port=4
  MotorNPConfig : Outport  Port=5
  tag scope: Bus_MotorParameters=global
  wires:
  MotorKv/1 -> Kv/1
  Product/1 -> Divide/1
  BatteryCapacityAh/1 -> Product/2
  BatteryCRating/1 -> Product/1
  MotorPhaseResistance/1 -> Bus Creator/1, PhaseResistance/1  "PhaseResistance"
  MotorPhaseInductance/1 -> Bus Creator/2, PhaseInductance/1  "PhaseInductance"
  MotorStatorTeeth/1 -> Vector Concatenate/1
  Vector Concatenate/1 -> MotorNPConfig/1
  NumberOfMotors/1 -> Divide/2
  Divide/1 -> MaxCurrentDraw/1
  Bus Creator/1 -> [Bus_MotorParameters]
  MotorPoles/1 -> Product1/1
  Product1/1 -> Vector Concatenate/2
  Constant/1 -> Product1/2

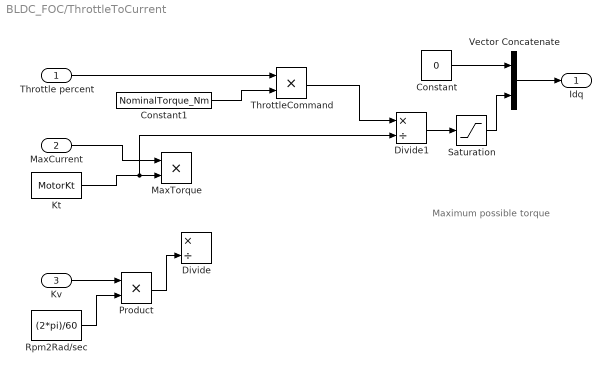
== system BLDC_FOC/ThrottleToCurrent ==
  note: Maximum possible torque
  Throttle percent : Inport
  MaxCurrent : Inport  Port=2
  Kv : Inport  Port=3
  Constant : Constant  Value=0
  Constant1 : Constant  Value=NominalTorque_Nm
  Divide : Product  Inputs=*/
  Divide1 : Product  Inputs=*/
  Kt : Constant  Value=MotorKt
  MaxTorque : Product  Inputs=**
  Product : Product
  Rpm2Rad/sec : Constant  Value=(2*pi)/60
  Saturation : Saturate  UpperLimit=MaxCurrentDraw  LowerLimit=0
  ThrottleCommand : Product
  Vector Concatenate : Concatenate
  Idq : Outport
  wires:
  Constant/1 -> Vector Concatenate/1
  Vector Concatenate/1 -> Idq/1
  Kv/1 -> Product/1
  Product/1 -> Divide/2
  Rpm2Rad/sec/1 -> Product/2
  Throttle percent/1 -> ThrottleCommand/1
  ThrottleCommand/1 -> Divide1/1
  Kt/1 -> Divide1/2, MaxTorque/2
  MaxCurrent/1 -> MaxTorque/1
  Constant1/1 -> ThrottleCommand/2
  Divide1/1 -> Saturation/1
  Saturation/1 -> Vector Concatenate/2

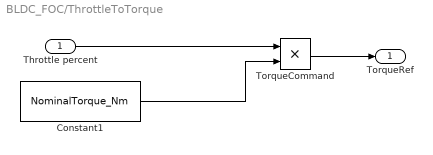
== system BLDC_FOC/ThrottleToTorque ==
  Throttle percent : Inport
  Constant1 : Constant  Value=NominalTorque_Nm
  TorqueCommand : Product
  TorqueRef : Outport
  wires:
  Constant1/1 -> TorqueCommand/2
  Throttle percent/1 -> TorqueCommand/1
  TorqueCommand/1 -> TorqueRef/1

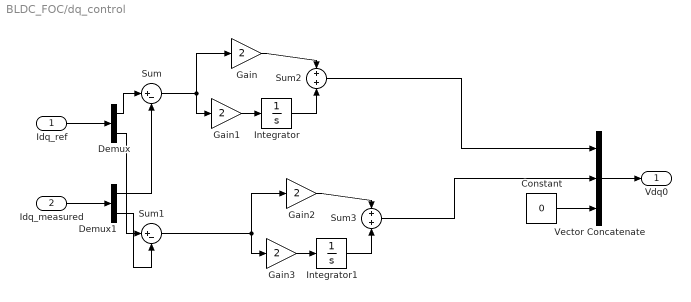
== system BLDC_FOC/dq_control ==
  Idq_ref : Inport
  Idq_measured : Inport  Port=2
  Constant : Constant  Value=0
  Demux : Demux  Outputs=2
  Demux1 : Demux  Outputs=2
  Gain{,1..3} (4 alike) : Gain  Gain=2
  Integrator : Integrator
  Integrator1 : Integrator
  Sum : Sum  Inputs=|+-
  Sum1 : Sum  Inputs=|+-
  Sum2 : Sum  Inputs=+|+
  Sum3 : Sum  Inputs=+|+
  Vector Concatenate : Concatenate  NumInputs=3
  Vdq0 : Outport
  wires:
  Vector Concatenate/1 -> Vdq0/1
  Constant/1 -> Vector Concatenate/3
  Idq_ref/1 -> Demux/1
  Demux/1 -> Sum/1
  Demux/2 -> Sum1/1
  Idq_measured/1 -> Demux1/1
  Demux1/1 -> Sum/2
  Demux1/2 -> Sum1/2
  Gain/1 -> Sum2/1
  Sum/1 -> Gain/1, Gain1/1
  Integrator/1 -> Sum2/2
  Gain1/1 -> Integrator/1
  Sum2/1 -> Vector Concatenate/1
  Gain3/1 -> Integrator1/1
  Integrator1/1 -> Sum3/2
  Sum1/1 -> Gain2/1, Gain3/1
  Gain2/1 -> Sum3/1
  Sum3/1 -> Vector Concatenate/2
